simulink model "a12_smlk"  (R2023b)
settings: Solver=ode45  StartTime=0.0  StopTime=2  RelTol=1e-3  EnableMultiTasking=on
values from neighbouring files (symbols this model uses):
  A = [-a-b  0  0 ... (first row only)    [a10_obs_contrls.m]    (also in a11_.m = [ 0   1; a12_.m = [ 0   1; a8_conversao_de_formas.m = [ 0  1; a8_state_space.m = [  0      1)
  alpha = inv((C-D*K)*inv(B*K-A)*B+D)    [a11_.m]    (also in a12_.m; a6_.m = 136.626132179)
  B = [ 1 ... (first row only)    [a10_obs_contrls.m]    (also in a11_.m = [ 0; a12_.m = [ 0; a8_conversao_de_formas.m = [ 0; a8_state_space.m = [ 0)
  C = [0 0 1]    [a10_obs_contrls.m]    (also in a11_.m = [ 1 0 ]; a12_.m = [ 1 0 ]; a3_exercicio.m = (s+2)/(s+1); a8_conversao_de_formas.m = [ 5  3 ])
  D = 0    [a11_.m]    (also in a12_.m; a5_sintonia.m = 1.2; a8_conversao_de_formas.m = 1; a8_state_space.m = [ 0 ])
  K = [ 102 19 ]    [a11_.m]    (also in a12_.m; a3_exercicio.m = 0.0938642036672; a4_exercicio.m = 0.2455; a5_sintonia.m = 23.8830609513)
  L = [ 39 ... (first row only)    [a12_.m]    (also in a3_exercicio.m = K*C*G; a9_exemplo_est_int.m = 1)
  r = 45    [a11_.m]    (also in a12_.m)
  x0 = [ 30 ... (first row only)    [a11_.m]    (also in a12_.m; a8_state_space.m = [ 1)
  X0 = [ 0 ... (first row only)    [a12_.m]
settings Model: Creator=andre.bergmann  LastModifiedBy=LUCAS
settings SolverCC: AlgebraicLoopSolver=TrustRegion
settings DataIOCC: LimitDataPoints=on  SaveFormat=Array  ReturnWorkspaceOutputs=off
settings OptimizationCC: ExpressionDepthLimit=2147483647  LifeSpan=inf
settings DebuggingCC: UnderspecifiedInitializationDetection=Classic  MergeDetectMultiDrivingBlocksExec=none  SolverPrmCheckMsg=warning  UnconnectedInputMsg=warning  UnconnectedOutputMsg=warning  UnconnectedLineMsg=warning  StateNameClashWarn=warning  SFUnexpectedBacktrackingDiag=warning  SFNoUnconditionalDefaultTransitionDiag=warning  SFExecutionAtInitializationDiag=none  ArithmeticOperatorsInVariantConditions=warning
settings HardwareCC: ProdBitPerPointer=32  ProdBitPerSizeT=32  ProdBitPerPtrDiffT=32  ProdLargestAtomicFloat=None  ProdIntDivRoundTo=Undefined  ProdEndianess=Unspecified  ProdWordSize=32  ProdHWDeviceType=32-bit Generic
settings ModelReferenceCC: PropagateSignalLabelsOutOfModel=off
settings SFSimCC: SimUseLocalCustomCode=off  CustomCodeUndefinedFunction=UseInterfaceOnly
settings RTWCC: RTWUseLocalCustomCode=off
settings CodeAppCC: StateflowObjectComments=on
settings GRTTargetCC: TargetLangStandard=C89/C90 (ANSI)
settings ConfigComp: CovMetricSettings=dw  CovSaveCumulativeToWorkspaceVar=on  CovSaveSingleToWorkspaceVar=on  CovExternalEMLEnable=off

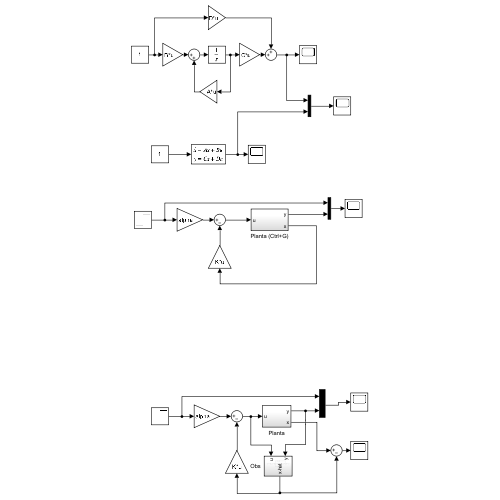
[thumbnail: Simulink's stored preview of the top-level diagram]
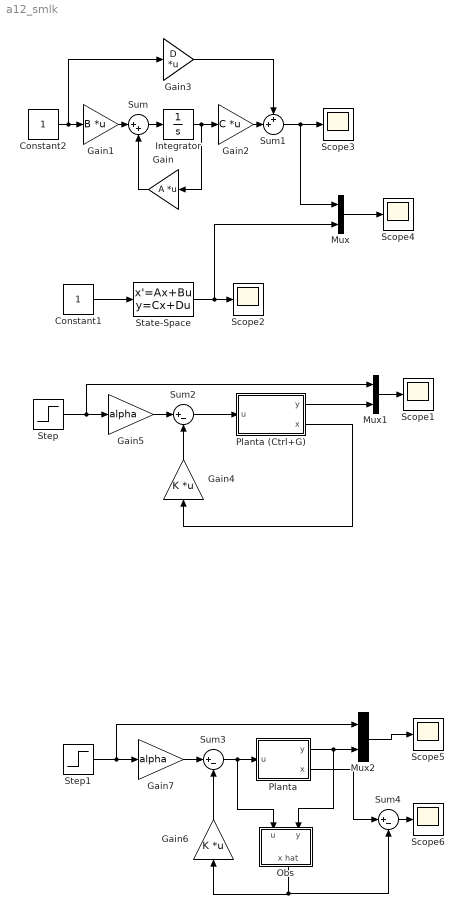
== system a12_smlk ==
  Constant1 : Constant
  Constant2 : Constant
  Gain : Gain  Gain=A  Multiplication=Matrix(K*u)
  Gain1 : Gain  Gain=B  Multiplication=Matrix(K*u)
  Gain2 : Gain  Gain=C  Multiplication=Matrix(K*u)
  Gain3 : Gain  Gain=D  Multiplication=Matrix(K*u)
  Gain4 : Gain  Gain=K  Multiplication=Matrix(K*u)
  Gain5 : Gain  Gain=alpha
  Gain6 : Gain  Gain=K  Multiplication=Matrix(K*u)
  Gain7 : Gain  Gain=alpha
  Integrator : Integrator  InitialCondition=x0
  Mux : Mux  Inputs=2
  Mux1 : Mux  Inputs=2
  Mux2 : Mux  Inputs=2
  Obs : Subsystem
  Planta : Subsystem
  Planta (Ctrl+G) : Subsystem
  Scope{1..6} (6 alike) : Scope
  State-Space : StateSpace  A=A  B=B  C=C  D=D  InitialCondition=x0
  Step : Step  After=r  SampleTime=0
  Step1 : Step  After=r  SampleTime=0
  Sum : Sum  Inputs=|++
  Sum1 : Sum  Inputs=++|
  Sum2 : Sum  Inputs=|+-
  Sum3 : Sum  Inputs=|+-
  Sum4 : Sum  Inputs=|+-
  wires:
  Sum2/1 -> Planta (Ctrl+G)/1(u)
  Planta (Ctrl+G)/1(y) -> Mux1/2
  Planta (Ctrl+G)/2(x) -> Gain4/1
  Constant1/1 -> State-Space/1
  State-Space/1 -> Mux/2, Scope2/1
  Constant2/1 -> Gain3/1, Gain1/1
  Gain/1 -> Sum/2
  Sum/1 -> Integrator/1
  Sum1/1 -> Mux/1, Scope3/1
  Gain2/1 -> Sum1/2
  Integrator/1 -> Gain2/1, Gain/1
  Gain3/1 -> Sum1/1
  Gain1/1 -> Sum/1
  Mux/1 -> Scope4/1
  Mux1/1 -> Scope1/1
  Gain4/1 -> Sum2/2
  Step/1 -> Mux1/1, Gain5/1
  Gain5/1 -> Sum2/1
  Step1/1 -> Mux2/1, Gain7/1
  Gain7/1 -> Sum3/1
  Mux2/1 -> Scope5/1
  Gain6/1 -> Sum3/2
  Sum3/1 -> Planta/1(u), Obs/1(u)
  Planta/1(y) -> Obs/2(y), Mux2/2
  Obs/1(x hat) -> Sum4/2, Gain6/1
  Planta/2(x) -> Sum4/1
  Sum4/1 -> Scope6/1

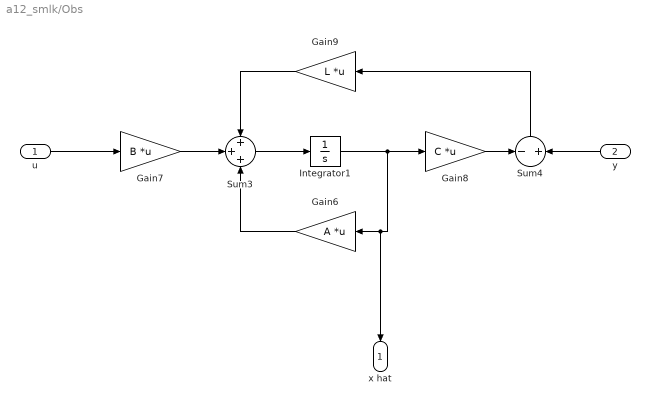
== system a12_smlk/Obs ==
  u : Inport
  y : Inport  Port=2
  Gain6 : Gain  Gain=A  Multiplication=Matrix(K*u)
  Gain7 : Gain  Gain=B  Multiplication=Matrix(K*u)
  Gain8 : Gain  Gain=C  Multiplication=Matrix(K*u)
  Gain9 : Gain  Gain=L  Multiplication=Matrix(K*u)
  Integrator1 : Integrator  InitialCondition=X0
  Sum3 : Sum  Inputs=+++
  Sum4 : Sum  Inputs=-|+
  x hat : Outport
  wires:
  Gain6/1 -> Sum3/3
  y/1 -> Sum4/2
  Integrator1/1 -> Gain6/1, x hat/1, Gain8/1
  Gain9/1 -> Sum3/1
  Sum3/1 -> Integrator1/1
  Gain7/1 -> Sum3/2
  Gain8/1 -> Sum4/1
  Sum4/1 -> Gain9/1
  u/1 -> Gain7/1

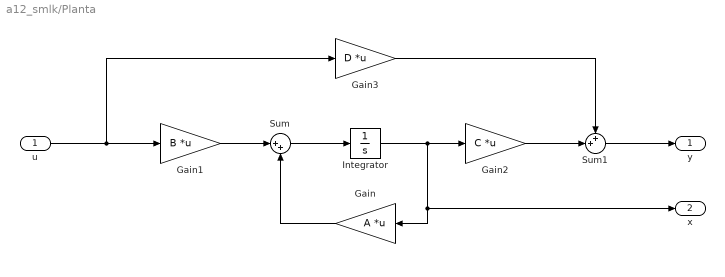
== system a12_smlk/Planta ==
  u : Inport
  Gain : Gain  Gain=A  Multiplication=Matrix(K*u)
  Gain1 : Gain  Gain=B  Multiplication=Matrix(K*u)
  Gain2 : Gain  Gain=C  Multiplication=Matrix(K*u)
  Gain3 : Gain  Gain=D  Multiplication=Matrix(K*u)
  Integrator : Integrator  InitialCondition=x0
  Sum : Sum  Inputs=|++
  Sum1 : Sum  Inputs=++|
  y : Outport
  x : Outport  Port=2
  wires:
  Gain1/1 -> Sum/1
  Gain2/1 -> Sum1/2
  u/1 -> Gain3/1, Gain1/1
  Sum1/1 -> y/1
  Sum/1 -> Integrator/1
  Gain3/1 -> Sum1/1
  Gain/1 -> Sum/2
  Integrator/1 -> x/1, Gain/1, Gain2/1

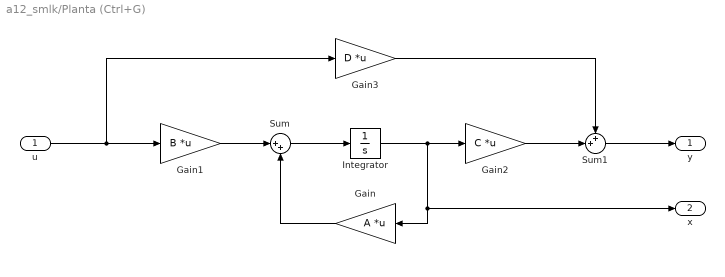
== system a12_smlk/Planta (Ctrl+G) ==
  u : Inport
  Gain : Gain  Gain=A  Multiplication=Matrix(K*u)
  Gain1 : Gain  Gain=B  Multiplication=Matrix(K*u)
  Gain2 : Gain  Gain=C  Multiplication=Matrix(K*u)
  Gain3 : Gain  Gain=D  Multiplication=Matrix(K*u)
  Integrator : Integrator  InitialCondition=x0
  Sum : Sum  Inputs=|++
  Sum1 : Sum  Inputs=++|
  y : Outport
  x : Outport  Port=2
  wires:
  Gain1/1 -> Sum/1
  Gain2/1 -> Sum1/2
  u/1 -> Gain3/1, Gain1/1
  Sum1/1 -> y/1
  Sum/1 -> Integrator/1
  Gain3/1 -> Sum1/1
  Gain/1 -> Sum/2
  Integrator/1 -> x/1, Gain/1, Gain2/1
